simulink model "rlwatertank"  (R2022a)
settings: Solver=ode45  StartTime=0.0  StopTime=inf  RelTol=1e-3  EnableMultiTasking=on
undefined symbols (not defined in the file): DiscIntNeverNeededParam
libraries: simulink x1, rllib x1
settings Model: Creator=sneha  LastModifiedBy=archi
settings SolverCC: AlgebraicLoopSolver=TrustRegion
settings DataIOCC: LimitDataPoints=on  SaveFormat=Array
settings OptimizationCC: LifeSpan=inf
settings DebuggingCC: UnconnectedInputMsg=warning  UnconnectedOutputMsg=warning  UnconnectedLineMsg=warning  SFUnexpectedBacktrackingDiag=warning  SFNoUnconditionalDefaultTransitionDiag=warning  SFExecutionAtInitializationDiag=none  SFMachineParentedDataDiag=warning  ArithmeticOperatorsInVariantConditions=warning
settings HardwareCC: ProdBitPerPointer=32  ProdBitPerSizeT=32  ProdBitPerPtrDiffT=32  ProdLargestAtomicFloat=None  ProdIntDivRoundTo=Undefined  ProdEndianess=Unspecified  ProdWordSize=32  ProdHWDeviceType=32-bit Generic
settings ModelReferenceCC: PropagateSignalLabelsOutOfModel=off
settings SFSimCC: SimUseLocalCustomCode=off  CustomCodeUndefinedFunction=UseInterfaceOnly
settings RTWCC: RTWUseLocalCustomCode=off
settings CodeAppCC: StateflowObjectComments=on
settings GRTTargetCC: TargetLangStandard=C89/C90 (ANSI)
settings ConfigComp: CovMetricSettings=dw  CovSaveCumulativeToWorkspaceVar=on  CovSaveSingleToWorkspaceVar=on  CovExternalEMLEnable=off

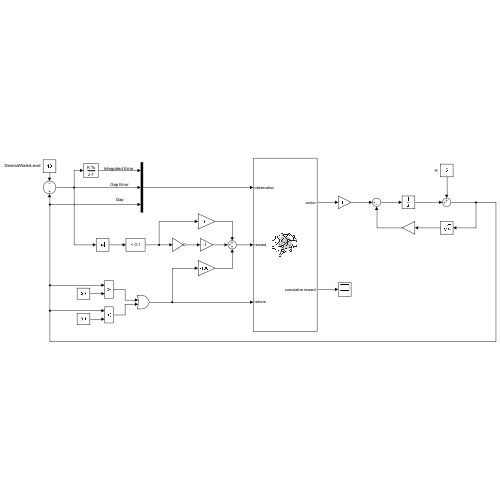
[thumbnail: Simulink's stored preview of the top-level diagram]
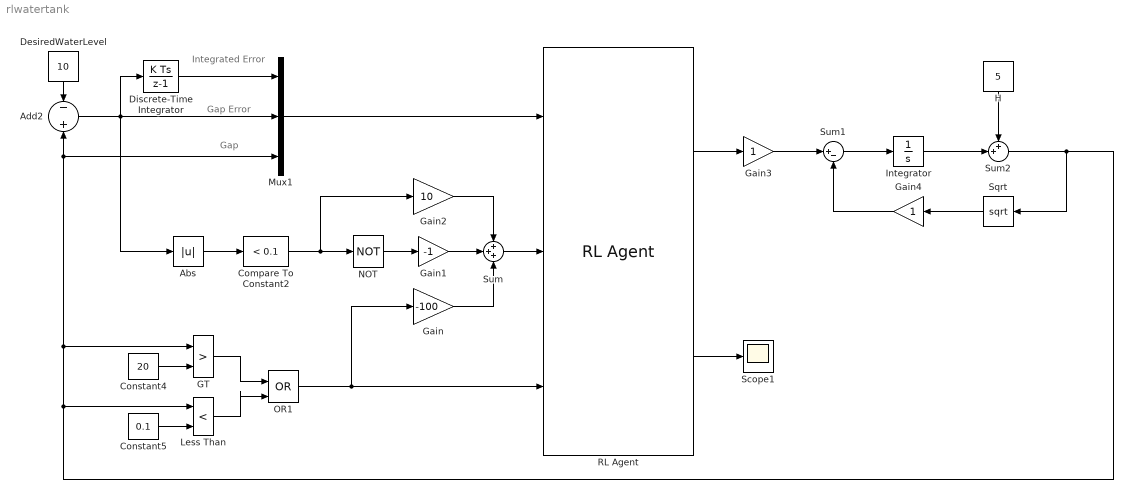
== system rlwatertank ==
  note: Gap
  note: Gap Error
  note: Integrated Error
  Abs : Abs  SaturateOnIntegerOverflow=off
  Add2 : Sum  Inputs=-|+
  Compare To Constant2 : simulink/Logic and Bit Operations/Compare To Constant  relop=<  const=0.1  OutDataTypeStr=boolean
  Constant4 : Constant  Value=20
  Constant5 : Constant  Value=0.1
  DesiredWaterLevel : Constant  Value=10
  Discrete-Time Integrator : DiscreteIntegrator  SampleTime=-1  ICPrevOutput=DiscIntNeverNeededParam  ICPrevScaledInput=DiscIntNeverNeededParam
  GT : RelationalOperator  Operator=>  OutDataTypeStr=boolean  RndMeth=Simplest  InputSameDT=off
  Gain : Gain  Gain=-100
  Gain1 : Gain  Gain=-1
  Gain2 : Gain  Gain=10
  Gain3 : Gain
  Gain4 : Gain
  H : Constant  Value=5
  Integrator : Integrator
  Less Than : RelationalOperator  Operator=<  OutDataTypeStr=boolean  RndMeth=Simplest  InputSameDT=off
  Mux1 : Mux  Inputs=3
  NOT : Logic  Operator=NOT  IconShape=distinctive  AllPortsSameDT=off  OutDataTypeStr=boolean
  OR1 : Logic  Operator=OR  IconShape=distinctive  AllPortsSameDT=off  OutDataTypeStr=boolean
  RL Agent : rllib/RL Agent  Agent=rlDDPGAgent  ExternalActionAsInput=off  ProvideLastAction=off  ProvideCumRwd=on  TreatAsDirectFeedthrough=on  UseStrictObservationDataTypes=off
  Scope1 : Scope
  Sqrt : Sqrt  OutputSignalType=real
  Sum : Sum  Inputs=+++
  Sum1 : Sum  Inputs=|+-
  Sum2 : Sum  Inputs=++|
  wires:
  RL Agent/2 -> Scope1/1
  DesiredWaterLevel/1 -> Add2/1
  Mux1/1 -> RL Agent/1
  Constant4/1 -> GT/2
  Integrator/1 -> Sum2/2
  Constant5/1 -> Less Than/2
  GT/1 -> OR1/1
  Less Than/1 -> OR1/2
  OR1/1 -> Gain/1, RL Agent/3
  Gain1/1 -> Sum/2
  Add2/1 -> Abs/1, Mux1/2, Discrete-Time Integrator/1
  Gain2/1 -> Sum/1
  NOT/1 -> Gain1/1
  Compare To Constant2/1 -> Gain2/1, NOT/1
  Gain/1 -> Sum/3
  Abs/1 -> Compare To Constant2/1
  Sum/1 -> RL Agent/2
  Discrete-Time Integrator/1 -> Mux1/1
  RL Agent/1 -> Gain3/1
  Gain3/1 -> Sum1/1
  Sum1/1 -> Integrator/1
  Gain4/1 -> Sum1/2
  Sqrt/1 -> Gain4/1
  H/1 -> Sum2/1
  Sum2/1 -> Sqrt/1, Less Than/1, GT/1, Mux1/3, Add2/2
